simulink model "x8"  (R2019b)
settings: Solver=VariableStepAuto  StartTime=0.0  StopTime=10.0  RelTol=1e-3
InitFcn:
  | parameters;
  | initialize;
undefined symbols (not defined in the file): state_init
settings Model: Creator=louis  LastModifiedBy=louis

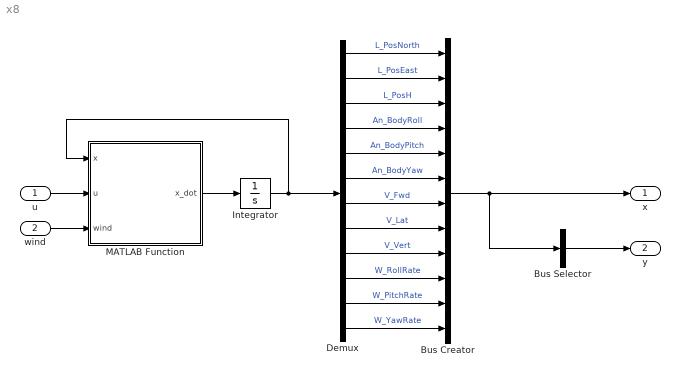
== system x8 ==
  u : Inport  PortDimensions=4
  wind : Inport  Port=2  PortDimensions=6
  Bus Creator : BusCreator  Inputs=12
  Bus Selector : BusSelector  OutputSignals=V_Fwd,An_BodyRoll,An_BodyPitch  OutputAsBus=on
  Demux : Demux  Outputs=12
  Integrator : Integrator  InitialCondition=state_init
  MATLAB Function : MATLAB Function  TreatAsAtomicUnit=on
  x : Outport
  y : Outport  Port=2
  wires:
  MATLAB Function/1(x_dot) -> Integrator/1
  u/1 -> MATLAB Function/2(u)
  wind/1 -> MATLAB Function/3(wind)
  Integrator/1 -> MATLAB Function/1(x), Demux/1
  Demux/1 -> Bus Creator/1  "L_PosNorth"
  Bus Creator/1 -> Bus Selector/1, x/1
  Demux/7 -> Bus Creator/7  "V_Fwd"
  Demux/2 -> Bus Creator/2  "L_PosEast"
  Demux/9 -> Bus Creator/9  "V_Vert"
  Demux/3 -> Bus Creator/3  "L_PosH"
  Demux/4 -> Bus Creator/4  "An_BodyRoll"
  Demux/8 -> Bus Creator/8  "V_Lat"
  Demux/10 -> Bus Creator/10  "W_RollRate"
  Demux/12 -> Bus Creator/12  "W_YawRate"
  Demux/11 -> Bus Creator/11  "W_PitchRate"
  Demux/5 -> Bus Creator/5  "An_BodyPitch"
  Demux/6 -> Bus Creator/6  "An_BodyYaw"
  Bus Selector/1 -> y/1

== matlab function x8/MATLAB Function ==
  data: x input; u input; x_dot output; wind input; P parameter
function x_dot = model(x,u,wind,P)

x_dot = dynamics(x,u,wind,P);

end
